simulink model "beta_estimator_acceleration"  (R2017a)
settings: Solver=VariableStepAuto  StartTime=0.0  StopTime=10.0  RelTol=1e-3
values from neighbouring files (symbols this model uses):
  N = 100    [taraPDscript.m]
undefined symbols (not defined in the file or in its folder): KD, KP
libraries: robotlib x3, simulink x2
settings Model: Creator=bascetta  LastModifiedBy=bascetta

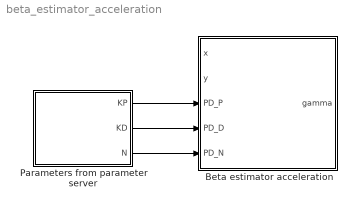
== system beta_estimator_acceleration ==
  Beta estimator acceleration : Subsystem
  Parameters from parameter server : Subsystem
  wires:
  Parameters from parameter server/3(N) -> Beta estimator acceleration/5(PD_N)
  Parameters from parameter server/2(KD) -> Beta estimator acceleration/4(PD_D)
  Parameters from parameter server/1(KP) -> Beta estimator acceleration/3(PD_P)

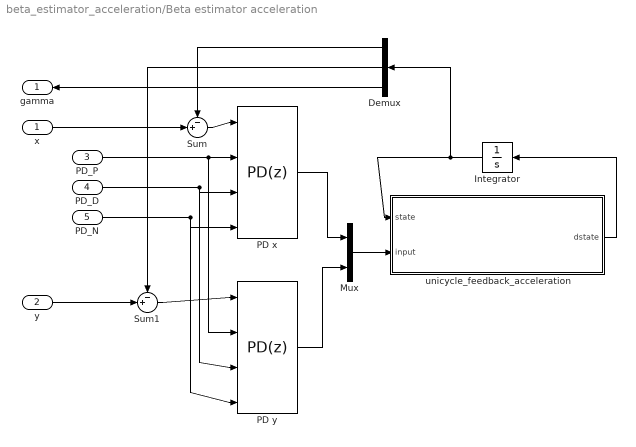
== system beta_estimator_acceleration/Beta estimator acceleration ==
  x : Inport
  y : Inport  Port=2
  PD_P : Inport  Port=3
  PD_D : Inport  Port=4
  PD_N : Inport  Port=5
  Demux : Demux  Outputs=3
  Integrator : Integrator
  Mux : Mux  Inputs=2
  PD x : simulink/Continuous/PID Controller  Controller=PD  TimeDomain=Discrete-time  SampleTime=-1  IntegratorMethod=Forward Euler  FilterMethod=Trapezoidal  Form=Parallel  UseFilter=on  ControllerParametersSource=external  P=KP  I=0  D=KD  N=N  InitialConditionSource=internal  InitialConditionForIntegrator=0  InitialConditionForFilter=0  ExternalReset=none  LimitOutput=off  UpperSaturationLimit=inf  LowerSaturationLimit=-inf  LinearizeAsGain=on  AntiWindupMode=none  Kb=1  TrackingMode=off  Kt=1  PParamMin=[]  PParamMax=[]  IParamMin=[]  IParamMax=[]  DParamMin=[]  DParamMax=[]  NParamMin=[]  NParamMax=[]  KbParamMin=[]  KbParamMax=[]  KtParamMin=[]  KtParamMax=[]  POutMin=[]  POutMax=[]  IOutMin=[]  IOutMax=[]  DOutMin=[]  DOutMax=[]  NOutMin=[]  NOutMax=[]  KbOutMin=[]  KbOutMax=[]  KtOutMin=[]  KtOutMax=[]  IntegratorOutMin=[]  IntegratorOutMax=[]  FilterOutMin=[]  FilterOutMax=[]  SumOutMin=[]  SumOutMax=[]  SumI1OutMin=[]  SumI1OutMax=[]  SumI2OutMin=[]  SumI2OutMax=[]  SumI3OutMin=[]  SumI3OutMax=[]  SumDOutMin=[]  SumDOutMax=[]  SaturationOutMin=[]  SaturationOutMax=[]  IntegratorContinuousStateAttributes=''  IntegratorStateMustResolveToSignalObject=off  IntegratorRTWStateStorageClass=Auto  FilterContinuousStateAttributes=''  FilterStateMustResolveToSignalObject=off  FilterRTWStateStorageClass=Auto  DifferentiatorICPrevScaledInput=0  DifferentiatorOutMin=[]  DifferentiatorOutMax=[]  InitialConditionSetting=State (most efficient)
  PD y : simulink/Continuous/PID Controller  Controller=PD  TimeDomain=Discrete-time  SampleTime=-1  IntegratorMethod=Forward Euler  FilterMethod=Trapezoidal  Form=Parallel  UseFilter=on  ControllerParametersSource=external  P=KP  I=0  D=KD  N=N  InitialConditionSource=internal  InitialConditionForIntegrator=0  InitialConditionForFilter=0  ExternalReset=none  LimitOutput=off  UpperSaturationLimit=inf  LowerSaturationLimit=-inf  LinearizeAsGain=on  AntiWindupMode=none  Kb=1  TrackingMode=off  Kt=1  PParamMin=[]  PParamMax=[]  IParamMin=[]  IParamMax=[]  DParamMin=[]  DParamMax=[]  NParamMin=[]  NParamMax=[]  KbParamMin=[]  KbParamMax=[]  KtParamMin=[]  KtParamMax=[]  POutMin=[]  POutMax=[]  IOutMin=[]  IOutMax=[]  DOutMin=[]  DOutMax=[]  NOutMin=[]  NOutMax=[]  KbOutMin=[]  KbOutMax=[]  KtOutMin=[]  KtOutMax=[]  IntegratorOutMin=[]  IntegratorOutMax=[]  FilterOutMin=[]  FilterOutMax=[]  SumOutMin=[]  SumOutMax=[]  SumI1OutMin=[]  SumI1OutMax=[]  SumI2OutMin=[]  SumI2OutMax=[]  SumI3OutMin=[]  SumI3OutMax=[]  SumDOutMin=[]  SumDOutMax=[]  SaturationOutMin=[]  SaturationOutMax=[]  IntegratorContinuousStateAttributes=''  IntegratorStateMustResolveToSignalObject=off  IntegratorRTWStateStorageClass=Auto  FilterContinuousStateAttributes=''  FilterStateMustResolveToSignalObject=off  FilterRTWStateStorageClass=Auto  DifferentiatorICPrevScaledInput=0  DifferentiatorOutMin=[]  DifferentiatorOutMax=[]  InitialConditionSetting=State (most efficient)
  Sum : Sum  Inputs=-+|
  Sum1 : Sum  Inputs=-+|
  unicycle_feedback_acceleration : MATLAB Function  TreatAsAtomicUnit=on
  gamma : Outport
  wires:
  unicycle_feedback_acceleration/1(dstate) -> Integrator/1
  Mux/1 -> unicycle_feedback_acceleration/2(input)
  Demux/1 -> Sum/1
  Sum1/1 -> PD y/1
  Sum/1 -> PD x/1
  PD x/1 -> Mux/1
  y/1 -> Sum1/2
  PD_P/1 -> PD y/2, PD x/2
  PD_N/1 -> PD y/4, PD x/4
  Demux/3 -> gamma/1
  PD_D/1 -> PD y/3, PD x/3
  Demux/2 -> Sum1/1
  x/1 -> Sum/2
  PD y/1 -> Mux/2
  Integrator/1 -> Demux/1, unicycle_feedback_acceleration/1(state)

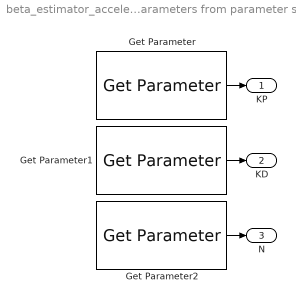
== system beta_estimator_acceleration/Parameters from parameter server ==
  Get Parameter : robotlib/Get Parameter  SourceLibraryInfo=This block requires Robotics System Toolbox  ParameterSource=Specify your own  ParameterName=/beta_estimator/KP  ParameterType=double  ParameterMaxArrayLength=16  ParameterInitialValue=0.0  SampleTime=-1  ShowErrorCodeOutput=off  ModelName=beta_estimator_acceleration  BlockId=ParamGet_beta_estimator_acceleration_22
      settings: SourceProductName=Robotics System Toolbox  SourceProductBaseCode=RO
  Get Parameter1 : robotlib/Get Parameter  SourceLibraryInfo=This block requires Robotics System Toolbox  ParameterSource=Specify your own  ParameterName=/beta_estimator/KD  ParameterType=double  ParameterMaxArrayLength=16  ParameterInitialValue=0.0  SampleTime=-1  ShowErrorCodeOutput=off  ModelName=beta_estimator_acceleration  BlockId=ParamGet_beta_estimator_acceleration_23
      settings: SourceProductName=Robotics System Toolbox  SourceProductBaseCode=RO
  Get Parameter2 : robotlib/Get Parameter  SourceLibraryInfo=This block requires Robotics System Toolbox  ParameterSource=Specify your own  ParameterName=/beta_estimator/N  ParameterType=double  ParameterMaxArrayLength=16  ParameterInitialValue=0.0  SampleTime=-1  ShowErrorCodeOutput=off  ModelName=beta_estimator_acceleration  BlockId=ParamGet_beta_estimator_acceleration_24
      settings: SourceProductName=Robotics System Toolbox  SourceProductBaseCode=RO
  KP : Outport
  KD : Outport  Port=2
  N : Outport  Port=3
  wires:
  Get Parameter1/1 -> KD/1
  Get Parameter2/1 -> N/1
  Get Parameter/1 -> KP/1

== matlab function beta_estimator_acceleration/Beta estimator acceleration/unicycle_feedback_acceleration ==
  data: state input; dstate output; input input
function dstate = unicycle_feedback_acceleration(state,input)

% State and input variables
x     = state(1);
y     = state(1);
gamma = state(3); % theta+beta
v     = state(4);
ax    = input(1);
ay    = input(2);

% Model equations
dstate = zeros(4,1);
dstate(1) = v*cos(gamma);
dstate(2) = v*sin(gamma);
dstate(3) = (ay*cos(gamma)-ax*sin(gamma))/v;
dstate(4) = ax*cos(gamma)+ay*sin(gamma);
